simulink model "amenl"  (Simulink 3.00)
settings: Solver=ode45  SolverMode=SingleTasking  StartTime=0.0  StopTime=100  MaxStep=0.10  RelTol=1e-4  AbsTol=1e-4
undefined symbols (not defined in the file or in its folder): dso, dsuo, nso, nsuo
settings Model: TimeSaveName=t  SaveOutput=off

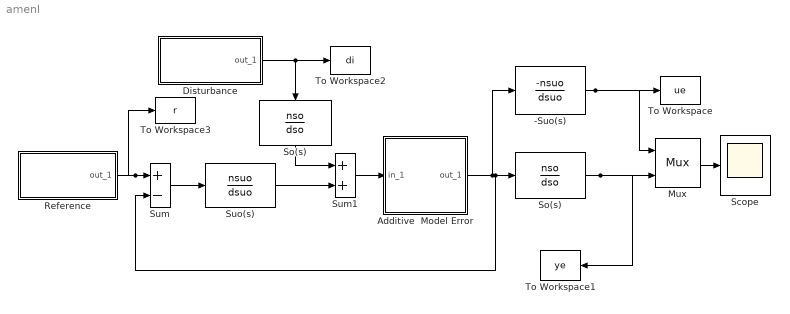
== system amenl ==
  -Suo(s) : TransferFcn  Numerator=-nsuo  Denominator=dsuo
      mask Type: SUO
      mask Display: disp('-Suo(s)')
  Additive  Model Error : Subsystem  mask(Additive modelling error){@1=nplin, @2=dplin}
      mask prompts: @1 "numerator linear model:"; @2 "denominator linear model:"
      mask help: Additive modelling error
      mask init:
      | nplin=@1;dplin=@2;
      mask Help: This block implements the AME for a non linear plant with modelling error
      mask Display: disp('AME')
  Disturbance : Subsystem  mask(Pulse disturbance){@1=1, @2=15, @3=30}
      mask prompts: @1 "pulse amplitude:"; @2 "initial time:"; @3 "pulse duration:"
      mask help: Pulse
      mask init:
      | D=@1;ti=@2;dt=@3;
      mask Help: This block generates a (one shot) pulse
      mask Display: disp('Disturbance')
  Mux : Mux  Inputs=2
      settings: DisplayOption=none
  Reference : Subsystem  mask(Reference){@1=2, @2=0.1, @3=0.3}
      mask prompts: @1 "average value:"; @2 "frequency square wave [rad/s]:"; @3 "peak value of square wave:"
      mask help: reference
      mask init:
      | Ro=@1;fsw=@2;asw=@3;
      mask Help: This block generates a signal with a mean value Ro and a superimposed square wave of frequency fsw [rad/s] and peak value asw.
      mask Display: disp('Reference')
  Scope : Scope
      settings: TickLabels=on  TimeRange=100.000000  YMin=-1  YMax=1  SaveToWorkspace=off  SaveName=ScopeData  DataFormat=Matrix
  So(s) : TransferFcn  Numerator=nso  Denominator=dso
      mask Type: SO
      mask Display: disp('So(s)')
  "So(s)  " : TransferFcn  Orientation=down  Numerator=nso  Denominator=dso
      mask Type: SO
      mask Display: disp('So(s)')
  Sum : Sum  Inputs=+-  SaturateOnIntegerOverflow=on
  Sum1 : Sum  Inputs=++  SaturateOnIntegerOverflow=on
  Suo(s) : TransferFcn  Numerator=nsuo  Denominator=dsuo
      mask Type: SUO
      mask Display: disp('Suo(s)')
  To Workspace : ToWorkspace  VariableName=ue  SampleTime=0  SaveFormat=Matrix
      settings: Buffer=20000
  To Workspace1 : ToWorkspace  VariableName=ye  SampleTime=0  SaveFormat=Matrix
      settings: Buffer=20000
  To Workspace2 : ToWorkspace  VariableName=di  SampleTime=0  SaveFormat=Matrix
      settings: Buffer=20000
  To Workspace3 : ToWorkspace  VariableName=r  SampleTime=0  SaveFormat=Matrix
      settings: Buffer=20000
  wires:
  Sum/1 -> Suo(s)/1
  Suo(s)/1 -> Sum1/2
  Sum1/1 -> Additive  Model Error/1(in_1)
  "So(s)  "/1 -> Sum1/1
  Additive  Model Error/1(out_1) -> -Suo(s)/1, So(s)/1, Sum/2
  Mux/1 -> Scope/1
  -Suo(s)/1 -> To Workspace/1, Mux/1
  Reference/1(out_1) -> Sum/1, To Workspace3/1
  So(s)/1 -> Mux/2, To Workspace1/1
  Disturbance/1(out_1) -> To Workspace2/1, "So(s)  "/1

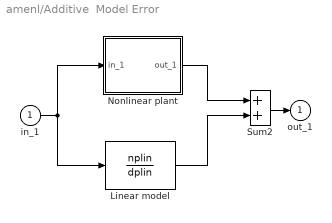
== system amenl/Additive  Model Error ==
  in_1 : Inport  Port=1  PortWidth=-1  SampleTime=-1  DataType=auto
      settings: SignalType=auto
  "Linear model " : TransferFcn  Numerator=nplin  Denominator=dplin
  Nonlinear plant : Subsystem
      mask Type: Real Plant
      mask Display: disp('Plant')
  Sum2 : Sum  Inputs=++  SaturateOnIntegerOverflow=on
  out_1 : Outport  Port=1  InitialOutput=0
  wires:
  in_1/1 -> Nonlinear plant/1(in_1), "Linear model "/1
  "Linear model "/1 -> Sum2/2
  Nonlinear plant/1(out_1) -> Sum2/1
  Sum2/1 -> out_1/1

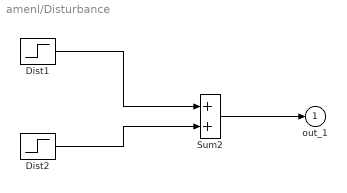
== system amenl/Disturbance ==
  Dist1 : Step  Time=ti  Before=0  After=D  SampleTime=0
  Dist2 : Step  Time=ti+dt  Before=0  After=-D  SampleTime=0
  Sum2 : Sum  Inputs=++  SaturateOnIntegerOverflow=on
  out_1 : Outport  Port=1  InitialOutput=0
  wires:
  Dist2/1 -> Sum2/2
  Dist1/1 -> Sum2/1
  Sum2/1 -> out_1/1

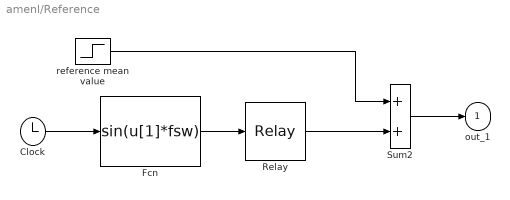
== system amenl/Reference ==
  Clock : Clock
      settings: DisplayTime=off  Decimation=10
  Fcn : Fcn  Expr=sin(u[1]*fsw)
  Relay : Relay  OnSwitchValue=0  OffSwitchValue=0  OnOutputValue=asw  OffOutputValue=-asw
  Sum2 : Sum  Inputs=++  SaturateOnIntegerOverflow=on
  reference mean value : Step  Time=0  Before=0  After=Ro  SampleTime=0
  out_1 : Outport  Port=1  InitialOutput=0
  wires:
  reference mean value/1 -> Sum2/1
  Sum2/1 -> out_1/1
  Clock/1 -> Fcn/1
  Fcn/1 -> Relay/1
  Relay/1 -> Sum2/2

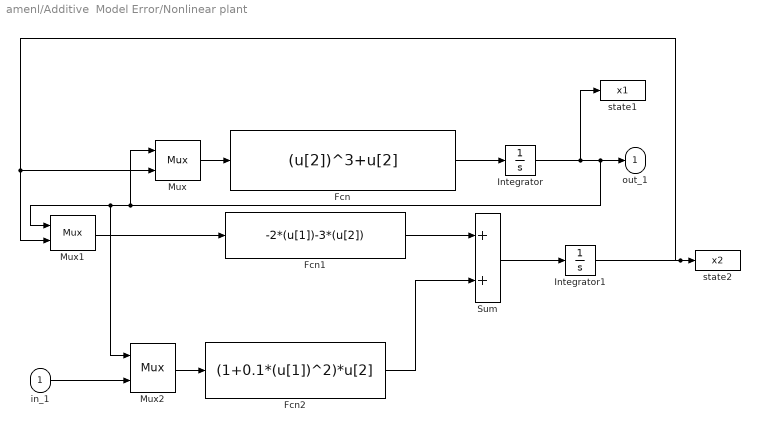
== system amenl/Additive  Model Error/Nonlinear plant ==
  in_1 : Inport  Port=1  PortWidth=-1  SampleTime=-1  DataType=auto
      settings: SignalType=auto
  Fcn : Fcn  Expr=(u[2])^3+u[2]
  Fcn1 : Fcn  Expr=-2*(u[1])-3*(u[2])
  Fcn2 : Fcn  Expr=(1+0.1*(u[1])^2)*u[2]
  Integrator : Integrator  ExternalReset=none  InitialConditionSource=internal  InitialCondition=0  LimitOutput=off  UpperSaturationLimit=inf  LowerSaturationLimit=-inf  ShowSaturationPort=off  ShowStatePort=off  AbsoluteTolerance=auto
  Integrator1 : Integrator  ExternalReset=none  InitialConditionSource=internal  InitialCondition=0  LimitOutput=off  UpperSaturationLimit=inf  LowerSaturationLimit=-inf  ShowSaturationPort=off  ShowStatePort=off  AbsoluteTolerance=auto
  Mux : Mux  Inputs=2
      settings: DisplayOption=none
  Mux1 : Mux  Inputs=2
      settings: DisplayOption=none
  Mux2 : Mux  Inputs=2
      settings: DisplayOption=none
  Sum : Sum  Inputs=++  SaturateOnIntegerOverflow=on
  state1 : ToWorkspace  VariableName=x1  SampleTime=0  SaveFormat=Matrix
      settings: Buffer=10000
  state2 : ToWorkspace  VariableName=x2  SampleTime=0  SaveFormat=Matrix
      settings: Buffer=10000
  out_1 : Outport  Port=1  InitialOutput=0
  wires:
  Integrator1/1 -> state2/1, Mux1/2, Mux/2
  Integrator/1 -> state1/1, out_1/1, Mux1/1, Mux2/1, Mux/1
  Mux2/1 -> Fcn2/1
  Fcn2/1 -> Sum/2
  Sum/1 -> Integrator1/1
  Fcn1/1 -> Sum/1
  Mux1/1 -> Fcn1/1
  Fcn/1 -> Integrator/1
  Mux/1 -> Fcn/1
  in_1/1 -> Mux2/2
